simulink model "PC_CONTROL_STATION"  (R2023b)
settings: Solver=FixedStepAuto  StartTime=0.0  StopTime=inf  RelTol=1e-3  EnableMultiTasking=on
InitFcn:
  | if RUN_MODE~=5
  |     % clear rpi;
  |     rpi = raspberrypi(CAR_IP, 'pi', 'LabControl');
  |     stopModel(rpi,'CAR_CONTROL_SYSTEM')
  |     while isModelRunning(rpi,'CAR_CONTROL_SYSTEM')
  |          stopModel(rpi,'CAR_CONTROL_SYSTEM')
  |     end
  |     runModel(rpi,'CAR_CONTROL_SYSTEM')
  |      while isModelRunning(rpi,'CAR_CONTROL_SYSTEM')==false
  |          runModel(rpi,'CAR_CONTROL_SYSTEM')
  |      end
  |      % clear rpi;
  | end
StopFcn:
  | if RUN_MODE~=5
  |    clear rpi;
  |    rpi = raspberrypi(CAR_IP, 'pi', 'LabControl');
  |    stopModel(rpi,'CAR_CONTROL_SYSTEM')
  |    while isModelRunning(rpi,'CAR_CONTROL_SYSTEM')
  |    end
  |    clear rpi;
  | end
model workspace (MAT data in the model file):
  SL_ROS_VariableLengthArrays_MaxSizes : object (value not decoded)
values from neighbouring files (symbols this model uses):
  data = theClient.GetLastFrameOfData()    [FuncMotive.m]
undefined symbols (not defined in the file or in its folder): CONTROL, CONTROL_INI, data_SL_Info, MD25, MSG, SAMPLING_TIME, Standard_Devices, SYSID_INPUT, TCP_Protocol, UDP_Protocol
libraries: simulink x51, sldrtlib x46, dspsigattribs x7, ros2lib x3, ctrlSharedLib x2, aerolibanimutils x1
(part 6 of 8)

== matlab function PC_CONTROL_STATION/PC TARGETS/PC TARGETS/NAVIGATION TARGETS/TRAJECTORY PLANNER (POLYNOMIAL IN Vx & Vy) ==
  data: CONTROL_IN input Bus: CONTROL_Bus; CONTROL output Bus: CONTROL_Bus
function CONTROL = MPC_TARGET_UPDATE(CONTROL_IN)

%--------------------------------------------------------------
% COPY CONTROL BUS
%--------------------------------------------------------------
CONTROL = CONTROL_IN;

%--------------------------------------------------------------
% DISABLING TARGET UPDATE
%--------------------------------------------------------------
% CONTROL_STATUS
% / 0. INITIALIZATION     / 1. ESTIMATION    / 2. ACTIVE CONTROL
if CONTROL.STATE.CONTROL_STATUS < 2  % INITIALIZATION    
    return
end

%--------------------------------------------------------------
% TIME MANAGEMENT
%--------------------------------------------------------------
% Sampling time 
ts = CONTROL.PARAM.SAMPLING_TIME;
% Trajectory update time 
tc = 10*ts;
persistent initialize TIMER
if isempty(initialize)
    TIMER = 0;
    initialize = 1;
end
TIMER = TIMER + ts;
if TIMER > tc-ts/2
    TIMER = 0;
    return
end

%--------------------------------------------------------------
% PARAMETERS
%--------------------------------------------------------------
% Maximun velocity magnitude 
VEL_MAG_MAX = CONTROL.PARAM.VEL_MAG_MAX;
% Prediction horizon (<= prediction horizon in mpcDesigner)
P = 20;
% Circular outline radius
% WP_R = CONTROL.PARAM.WP_R;

%--------------------------------------------------------------
% MEASUREMENTS AND STATE
%--------------------------------------------------------------
VEL_MAG = CONTROL.INPUT.FORWARD_VEL;
VEL_ANG = CONTROL.INPUT.YAW_ANG;
VEL_X = CONTROL.INPUT.EARTH_VEL(1);
VEL_Y = CONTROL.INPUT.EARTH_VEL(2);
POS_XY = CONTROL.INPUT.EARTH_POS(1:2);
WP_XY = CONTROL.PARAM.WP_XY;
NEXT_WP = CONTROL.STATE.NEXT_WP;
M = CONTROL.PARAM.NAV_MPC.PRED_HRZ;
if NEXT_WP == size(WP_XY,2)
    CONTROL.TARGET.NAV_REF_LC(1) = 0;
    CONTROL.TARGET.NAV_REF(1) = 0;
    CONTROL.TARGET.NAV_REF_MPC(1:M,1) = zeros(M,1);
    CONTROL.TARGET.VEL_XY_REF(1) = 0;
    CONTROL.TARGET.VEL_XY_REF(2) = 0;
    CONTROL.TARGET.FORWARD_VEL_REF = 0;
end

%--------------------------------------------------------------
% TRAJECTORY PLANNING
%--------------------------------------------------------------
% x(t) = sum(ai*t^i) i=0...N
% y(t) = sum(bi*t^i) i=0...N
% dx(t)/dt = vx(t) = sum(i*ai*t^(i-1)) i=0...N
% dy(t)/dt = vy(t) = sum(i*bi*t^(i-1)) i=0...N
% Position and distance data
pos_x = [POS_XY(1) WP_XY(1,NEXT_WP:end)]';
pos_y = [POS_XY(2) WP_XY(2,NEXT_WP:end)]'; 
d = abs(diff(pos_x) + 1j*diff(pos_y));
% Delete duplicated points (distance = 0)
ind = find(d>0);
pos_x = [pos_x(ind) ; pos_x(end)];
pos_y = [pos_y(ind) ; pos_y(end)];
d = abs(diff(pos_x) + 1j*diff(pos_y));
% Polynomial parameters
Np = min([4 length(pos_x)+1]);
% Polynomial order
N = Np-1;
% Parameter initialization
a = zeros(Np,1);
b = zeros(Np,1);
a(1) = pos_x(1);
b(1) = pos_y(1);
a(2) = VEL_X;
b(2) = VEL_Y;
% Time vector for target
t_tgt = (1:P)'*tc;
VEL_MAG_TARGET = zeros(P,1);
VEL_ANG_TARGET = zeros(P,1);
% Time matrix for velocity target computation
matTp = zeros(P,N+1);
matTv = zeros(P,N);
for nn = 1:N+1
    matTp(:,nn) = t_tgt.^(nn-1);
end
for nn = 1:N
    matTv(:,nn) = nn*t_tgt.^(nn-1);
end
flag_vel_max = true;
k = 1;
while flag_vel_max
    % Reaching time for the next waypoints
    t = cumsum([0 ; k*sqrt(2)*d(1:N-1)/VEL_MAG_MAX]);    
    % Polynomial coefficient estimation 
    % matBx = matA*a(3:Np);  
    % matBy = matA*b(3:Np)
    matA = zeros(Np-2);
    for nn = 1:Np-2
        matA(:,nn) = t(2:end).^(nn+1);
    end
    matBx = pos_x(2:Np-1) - a(2)*t(2:end) - a(1);
    matBy = pos_y(2:Np-1) - b(2)*t(2:end) - b(1);
    inv_matA = inv(matA);
    a(3:end) = inv_matA*matBx;
    b(3:end) = inv_matA*matBy;
    % Position target calculation
    px_tgt = matTp*a;
    py_tgt = matTp*b; 
    % Magnitude and angle velocity targets calculation
    vx_tgt = matTv*a(2:end);
    vy_tgt = matTv*b(2:end); 
    v_tgt = vx_tgt + 1j*vy_tgt;
    VEL_MAG_TARGET = abs(v_tgt);
    VEL_ANG_TARGET = angle(v_tgt)*(VEL_MAG_TARGET(1)>=0.005) + ...
                    VEL_ANG*ones(size(VEL_ANG_TARGET))*(VEL_MAG_TARGET(1)<0.005);
    % Decreasing velocity factor
    k = k*max(VEL_MAG_TARGET)/VEL_MAG_MAX;
    % Maximun velocity verification
    if (max(VEL_MAG_TARGET)/VEL_MAG_MAX)<=1.01
        flag_vel_max = false;
    end
end

%--------------------------------------------------------------
% UNWRAPPING
%--------------------------------------------------------------
aux1 = VEL_ANG_TARGET(1);
aux2 = VEL_ANG;
INC_VEL_ANG_TARGET = zeros(21,1);
INC_VEL_ANG_TARGET(1) = aux1-aux2;
for nn=1:10
    INC_VEL_ANG_TARGET(2*nn:2*nn+1) = [aux1-aux2-2*nn*pi ; aux1-aux2+2*nn*pi];
end
[~,ind] = min(abs(INC_VEL_ANG_TARGET));
VEL_ANG_TARGET(1) = aux2 + INC_VEL_ANG_TARGET(ind);
for nn = 2:P
    INC_VEL_ANG_TARGET = [VEL_ANG_TARGET(nn)-VEL_ANG_TARGET(nn-1)
                          VEL_ANG_TARGET(nn)-VEL_ANG_TARGET(nn-1)-2*pi
                          VEL_ANG_TARGET(nn)-VEL_ANG_TARGET(nn-1)+2*pi];
    [~,ind] = min(abs(INC_VEL_ANG_TARGET));
    VEL_ANG_TARGET(nn) = VEL_ANG_TARGET(nn-1) + INC_VEL_ANG_TARGET(ind);
end

%--------------------------------------------------------------
% CONTROL BUS UPDATE
%--------------------------------------------------------------
CONTROL.TARGET.NAV_REF_LC(1) = VEL_MAG_TARGET(1);
CONTROL.TARGET.NAV_REF_LC(2) = VEL_ANG_TARGET(1);
if M<=P
    CONTROL.TARGET.NAV_REF_MPC(1:M,1) = VEL_MAG_TARGET(1:M);
    CONTROL.TARGET.NAV_REF_MPC(1:M,2) = VEL_ANG_TARGET(1:M);
else
    CONTROL.TARGET.NAV_REF_MPC(1:M,1) = [VEL_MAG_TARGET(1:P); VEL_MAG_TARGET(end)*ones(M-P,1)];
    CONTROL.TARGET.NAV_REF_MPC(1:M,2) = [VEL_ANG_TARGET(1:P); VEL_ANG_TARGET(end)*ones(M-P,1)];
end
VEL_XY = VEL_MAG_TARGET.*exp(1j*VEL_ANG_TARGET);
CONTROL.TARGET.VEL_XY_REF(1) = real(VEL_XY(1));
CONTROL.TARGET.VEL_XY_REF(2) = imag(VEL_XY(1));
CONTROL.TARGET.FORWARD_VEL_REF = VEL_MAG_TARGET(1);
CONTROL.TARGET.YAW_ANG_REF = VEL_ANG_TARGET(1);
CONTROL.TARGET.NAV_REF = [CONTROL.TARGET.FORWARD_VEL_REF ; CONTROL.TARGET.YAW_ANG_REF];

return

== matlab function PC_CONTROL_STATION/PC TARGETS/PC TARGETS/WFL TARGETS/ PULSE GENERATION ==
  data: CONTROL input Bus: CONTROL_Bus; WALL_DIST_REF output
function WALL_DIST_REF = PULSE_GEN(CONTROL)
    
persistent TIMER initialize
if isempty(initialize)
    TIMER = 0;
    initialize = 1;
end

% SAMPLING TIME
SAMPLING_TIME = CONTROL.PARAM.SAMPLING_TIME; % s

%% OPERATION MODE
% / 0. BOOTING   / 1. SENSOR CALIBRATION / 2. READY
% / 3. OPEN LOOP / 4. ATTITUDE / 5. VELOCITY / 6. NAVIGATION / 
% / 7. WALL FOLLOWER / 8. WALL-FOLLOWER COMPETITION / 
% / 9. NAVIGATION COMPETITION / 10. STOP
CURRENT_STATUS = CONTROL.STATE.CURRENT_STATUS_SYS;
PREVIOUS_STATUS = CONTROL.STATE.PREVIOUS_STATUS;

if (CURRENT_STATUS == 7) && (PREVIOUS_STATUS == 7)   
    if TIMER > 15
        WALL_DIST_REF = 0.1;
    elseif TIMER < 5
        WALL_DIST_REF = 0.1;
        TIMER = TIMER + SAMPLING_TIME;
    else % 5 <= TIMER <= 15
        WALL_DIST_REF = 0.125;
        TIMER = TIMER + SAMPLING_TIME;
    end
else
    WALL_DIST_REF = 0.1;
    TIMER = 0;
end

== matlab function PC_CONTROL_STATION/MONITORING/SYSTEM IDENTIFICATION/Second-order equation ==
  data: b input; r1 output; c input; r2 output
function [r1,r2] = sol_2ord_eq(b,c)
r1 = (-b+sqrt(abs(b^2-4*c)))/2;
r2 = (-b-sqrt(abs(b^2-4*c)))/2;
return
